simulink model "PID_controller_long_stage2"  (R2019a)
settings: Solver=VariableStepAuto  StartTime=0.0  StopTime=5  FixedStep=1e-3  RelTol=1e-5
undefined symbols (not defined in the file): sys
libraries: aerolibactuator x1, simulink x1
settings Model: Creator=tyson  LastModifiedBy=tyson
settings DebuggingCC: InheritedTsInSrcMsg=none

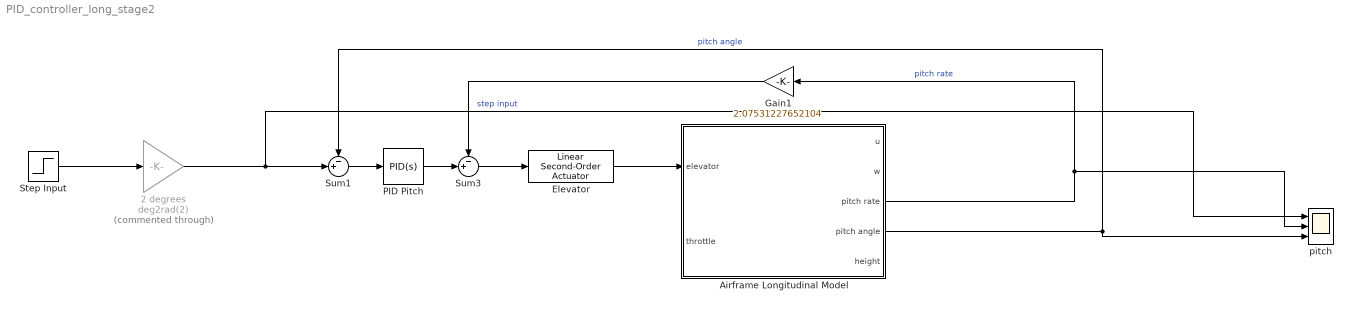
== system PID_controller_long_stage2 ==
  2 degrees : Gain  Commented=through  Gain=deg2rad(2)
  Airframe Longitudinal Model : Subsystem
      mask Display: image('/home/tyson/Dropbox/Academic/4th Year/ELEN4011/matlab/icons/airframe_long.png');
  Elevator : aerolibactuator/Linear Second-Order Actuator  wn_fin=actuators.naturalFreq  z_fin=actuators.dampingRatio  fin_act_0=0  fin_act_vel=0
      settings: SourceProductName=Aerospace Blockset  SourceProductBaseCode=AE
  Gain1 : Gain  Gain=2.07531227652104
  PID Pitch : simulink/Continuous/PID Controller  Controller=PID  Form=Parallel  TimeDomain=Continuous-time  SampleTime=-1  IntegratorMethod=Forward Euler  FilterMethod=Forward Euler  ControllerParametersSource=internal  P=11.8511840404623  I=5.20528630472053  D=6.6250954156956  UseFilter=on  N=51.2657243257402  TunerSelectOption=Transfer Function Based (PID Tuner App)  InitialConditionSource=internal  InitialConditionForIntegrator=0  InitialConditionForFilter=0  DifferentiatorICPrevScaledInput=0  ExternalReset=none  TrackingMode=off  Kt=1  LimitOutput=off  UpperSaturationLimit=inf  LowerSaturationLimit=-inf  LinearizeAsGain=on  AntiWindupMode=none  Kb=1  POutMin=[]  POutMax=[]  IOutMin=[]  IOutMax=[]  DOutMin=[]  DOutMax=[]  NOutMin=[]  NOutMax=[]  SumOutMin=[]  SumOutMax=[]  SaturationOutMin=[]  SaturationOutMax=[]  PParamMin=[]  PParamMax=[]  IParamMin=[]  IParamMax=[]  DParamMin=[]  DParamMax=[]  NParamMin=[]  NParamMax=[]  KbParamMin=[]  KbParamMax=[]  KtParamMin=[]  KtParamMax=[]  KbOutMin=[]  KbOutMax=[]  KtOutMin=[]  KtOutMax=[]  IntegratorOutMin=[]  IntegratorOutMax=[]  FilterOutMin=[]  FilterOutMax=[]  SumI1OutMin=[]  SumI1OutMax=[]  SumI2OutMin=[]  SumI2OutMax=[]  SumI3OutMin=[]  SumI3OutMax=[]  SumI4OutMin=[]  SumI4OutMax=[]  SumDOutMin=[]  SumDOutMax=[]  DifferentiatorOutMin=[]  DifferentiatorOutMax=[]  FilterDiffOutCoefMin=[]  FilterDiffOutCoefMax=[]  ReciprocalOutMin=[]  ReciprocalOutMax=[]  SumDenOutMin=[]  SumDenOutMax=[]  SumNumOutMin=[]  SumNumOutMax=[]  DivideOutMin=[]  DivideOutMax=[]  IntegratorContinuousStateAttributes=''  IntegratorStateMustResolveToSignalObject=off  IntegratorRTWStateStorageClass=Auto  FilterContinuousStateAttributes=''  FilterStateMustResolveToSignalObject=off  FilterRTWStateStorageClass=Auto  ParallelPVariant=InternalParameters  IdealPVariant=Disabled  IVariant=InternalParameters  DVariant=InternalParameters  IntegratorVariant=Continuous  SatVariant=Disabled  AWVariant=Passthrough  PCopyVariant=Disabled  TRVariant=Disabled  FdbkBlocksVariant=Forward  IdealPFdbkVariant=Disabled  SatFdbkVariant=Disabled  DerivativeFilterVariant=ContFilter  NVariant=InternalParameters  NCopyVariant=Disabled  FilterICVariant=InternalICsFilter  IntegratorICVariant=InternalICs  ExternalResetVariant=Disabled  TRSumVariant=Passthrough  SumFdbkVariant=Disabled  SumVariant=Sum_PID
  Step Input : Step
  Sum1 : Sum  Inputs=-+|
  Sum3 : Sum  Inputs=-+|
  pitch : Scope  NumInputPorts=3
  wires:
  Airframe Longitudinal Model/4(pitch angle) -> Sum1/1, pitch/3  "pitch angle"
  Elevator/1 -> Airframe Longitudinal Model/1(elevator)
  Sum1/1 -> PID Pitch/1
  PID Pitch/1 -> Sum3/2
  Step Input/1 -> 2 degrees/1
  Sum3/1 -> Elevator/1
  Gain1/1 -> Sum3/1
  Airframe Longitudinal Model/3(pitch rate) -> pitch/2, Gain1/1  "pitch rate"
  2 degrees/1 -> pitch/1, Sum1/2  "step input"

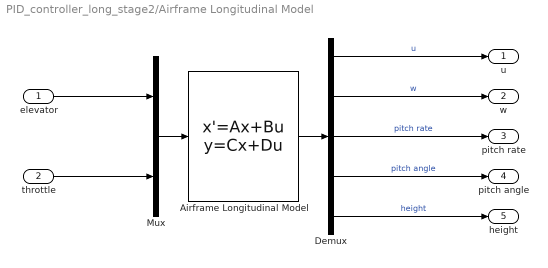
== system PID_controller_long_stage2/Airframe Longitudinal Model ==
  elevator : Inport
  throttle : Inport  Port=2
  Airframe Longitudinal Model : StateSpace  A=sys.long.A  B=sys.long.B  C=sys.long.C  D=sys.long.D  InitialCondition=0
  Demux : Demux  Outputs=5
  Mux : Mux  Inputs=2
  u : Outport
  w : Outport  Port=2
  pitch rate : Outport  Port=3
  pitch angle : Outport  Port=4
  height : Outport  Port=5
  wires:
  throttle/1 -> Mux/2
  Demux/4 -> pitch angle/1  "pitch angle"
  Demux/3 -> pitch rate/1  "pitch rate"
  Mux/1 -> Airframe Longitudinal Model/1
  Airframe Longitudinal Model/1 -> Demux/1
  Demux/1 -> u/1  "u"
  Demux/2 -> w/1  "w"
  Demux/5 -> height/1  "height"
  elevator/1 -> Mux/1
